simulink model "ROPOD_Control_WheelsRL_Code_GEN"  (R2020b)
settings: Solver=VariableStepAuto  StartTime=0.0  StopTime=10.0  RelTol=1e-3
values from neighbouring files (symbols this model uses):
  FFtheta_intia = 0    [init_model.m]
  FFxy_mass = 0*80    (= 0)    [init_model.m]
  I_fhz_ddelta_cntr = 0    [init_model.m]
  I_fhz_dtheta_cntr = 0.3    [init_model.m]
  I_fhz_dxdy_cntr = 0.25    [init_model.m]
  K_gain_ddelta_cntr = 0.2    [init_model.m]
  K_gain_dtheta_cntr = 150    [init_model.m]
  K_gain_dxdy_cntr = 200    [init_model.m]
  LL_wp_fhz_ddelta_cntr = 10    [init_model.m]
  LL_wp_fhz_dtheta_cntr = 20    [init_model.m]
  LL_wp_fhz_dxdy_cntr = 20    [init_model.m]
  LL_wz_fhz_ddelta_cntr = 2    [init_model.m]
  LL_wz_fhz_dtheta_cntr = 20    [init_model.m]
  LL_wz_fhz_dxdy_cntr = 20    [init_model.m]
  LPF_fhz_ddelta_cntr = 10    [init_model.m]
  LPF_fhz_ddelta_meas = 50    [init_model.m]
  LPF_fhz_dtheta_cntr = 100    [init_model.m]
  LPF_fhz_dvarphi_meas = 50    [init_model.m]
  LPF_fhz_dxdy_cntr = 100    [init_model.m]
  max_hw_tau = 7.0    (= 7)    [init_model.m]
  max_ropod_acc_theta = 1.6    [init_model.m]
  max_ropod_acc_xy = 2.0    (= 2)    [init_model.m]
  max_ropod_sw_force = 500    [init_model.m]
  max_ropod_sw_tau = 250    [init_model.m]
  max_ropod_vel_theta = 1.6    [init_model.m]
  max_ropod_vel_xy = 2.0    (= 2)    [init_model.m]
  max_sw_current = 10    [init_model.m]
  Nwheels = 4    [Jqwl_numeric_function.m]    (also in S_matrix.m; extract_kinmodel_parameters.m; init_model.m; tau_optimal_dist_vec_fun.m)
  pivot_offs_sws = [3.835 3.465 2.059 0.357]    [init_model.m]
  ropod_kinmodel_pv = struct2array(ropod_kinmodel_param)    [set_ropod_KinModparams.m]
  SW_COM1_ENABLE1 = hex2dec('0001')    [init_model.m]
  SW_COM1_ENABLE2 = hex2dec('0002')    [init_model.m]
  SW_COM1_MODE_TORQUE = bitshift(hex2dec('0000'),2)    [init_model.m]
  SW_COM1_MODE_VELOCITY = bitshift(hex2dec('0002'),2)    [init_model.m]
  SW_COM1_USE_TS = hex2dec('8000')    [init_model.m]
  Tinit = 0*Tslot    [init_model.m]
  Ts = 0.001    [init_model.m]
undefined symbols (not defined in the file or in its folder): AgentNumber, DiscIntNeverNeededParam, flock_FFtheta_friction, flock_FFxy_friction, I_fhz_dtheta_flock_cntr, I_fhz_dvarphi_cntr, I_fhz_dxdy_flock_cntr, K_gain_dtheta_flock_cntr, K_gain_dvarphi_cntr, K_gain_dxdy_flock_cntr, LL_wp_fhz_dtheta_flock_cntr, LL_wp_fhz_dvarphi_cntr, LL_wp_fhz_dxdy_flock_cntr, LL_wz_fhz_dtheta_flock_cntr, LL_wz_fhz_dvarphi_cntr, LL_wz_fhz_dxdy_flock_cntr, LPF_fhz_dtheta_flock_cntr, LPF_fhz_dvarphi_cntr, LPF_fhz_dxdy_flock_cntr, max_flock_acc_theta, max_flock_acc_xy, max_flock_vel_theta, max_flock_vel_xy, Nagents, ropod_position_inflock, sw_tau_2_current, Tsflck
libraries: simulink x62, pid_lib x60, cstblocks x54, dspsigops x24, SOEM_EtherCAT_Lib x5, dspnetwork x4
(part 10 of 11)

== system ROPOD_Control_WheelsRL_Code_GEN/RopodTorqueDistribution_/wheel vel cntr/Wheels Velocity controller/G_I_LL_LPF Controller7/Shapeit Integrator (Tustin) ==
  In : Inport
  I_fhz : Inport  Port=2
  reset : Inport  Port=3
  Constant : Constant  Value=0
  Constant4 : Constant
  Constant5 : Constant  Value=0
  Gain2 : Gain  Gain=2*pi
  PID Controller3 : pid_lib/PID Controller  Controller=PID  Form=Parallel  TimeDomain=Discrete-time  UseExternalTs=off  SampleTime=Ts  IntegratorMethod=Trapezoidal  FilterMethod=Trapezoidal  ControllerParametersSource=external  P=0.4  I=0.4*2*pi*3  D=0  UseFilter=on  N=100  TunerSelectOption=Transfer Function Based (PID Tuner App)  InitialConditionSource=internal  InitialConditionForIntegrator=0  InitialConditionForFilter=0  DifferentiatorICPrevScaledInput=0  ExternalReset=level  TrackingMode=off  Kt=1  LimitOutput=on  SatLimitsSource=internal  UpperSaturationLimit=max_hw_tau  LowerSaturationLimit=-max_hw_tau  LinearizeAsGain=on  AntiWindupMode=clamping  Kb=1  POutMin=[]  POutMax=[]  IOutMin=[]  IOutMax=[]  DOutMin=[]  DOutMax=[]  NOutMin=[]  NOutMax=[]  SumOutMin=[]  SumOutMax=[]  SaturationOutMin=[]  SaturationOutMax=[]  PParamMin=[]  PParamMax=[]  IParamMin=[]  IParamMax=[]  DParamMin=[]  DParamMax=[]  NParamMin=[]  NParamMax=[]  KbParamMin=[]  KbParamMax=[]  KtParamMin=[]  KtParamMax=[]  KbOutMin=[]  KbOutMax=[]  KtOutMin=[]  KtOutMax=[]  IntegratorOutMin=[]  IntegratorOutMax=[]  FilterOutMin=[]  FilterOutMax=[]  SumI1OutMin=[]  SumI1OutMax=[]  SumI2OutMin=[]  SumI2OutMax=[]  SumI3OutMin=[]  SumI3OutMax=[]  SumI4OutMin=[]  SumI4OutMax=[]  SumDOutMin=[]  SumDOutMax=[]  DifferentiatorOutMin=[]  DifferentiatorOutMax=[]  FilterDiffOutCoefMin=[]  FilterDiffOutCoefMax=[]  ReciprocalOutMin=[]  ReciprocalOutMax=[]  SumDenOutMin=[]  SumDenOutMax=[]  SumNumOutMin=[]  SumNumOutMax=[]  DivideOutMin=[]  DivideOutMax=[]  UdiffTsProdOutMin=[]  UdiffTsProdOutMax=[]  NTsProdOutMin=[]  NTsProdOutMax=[]  UintegralTsProdOutMin=[]  UintegralTsProdOutMax=[]  UngainTsProdOutMin=[]  UngainTsProdOutMax=[]  IntegratorContinuousStateAttributes=''  IntegratorStateMustResolveToSignalObject=off  IntegratorRTWStateStorageClass=Auto  FilterContinuousStateAttributes=''  FilterStateMustResolveToSignalObject=off  FilterRTWStateStorageClass=Auto  ParallelPVariant=ExternalParameters  IdealPVariant=Disabled  IVariant=ExternalParameters  DVariant=ExternalParameters  IntegratorVariant=Discrete  SatVariant=Enabled  AWVariant=DiscClampingParallel  PCopyVariant=Disabled  TRVariant=Disabled  FdbkBlocksVariant=Feedback  IdealPFdbkVariant=Passthrough  SatFdbkVariant=Passthrough  DerivativeFilterVariant=TrapezoidalFilter  NVariant=ExternalParameters  NCopyVariant=ExternalParameters  FilterICVariant=InternalICsFilter  IntegratorICVariant=InternalICs  ExternalResetVariant=ExternalReset  TRSumVariant=Passthrough  SumFdbkVariant=Enabled  SumVariant=Sum_PID  TsampFilterVariant=InternalTs  TsampNgainVariant=Passthrough  TsampIntegralVariant=Passthrough  ExternalSaturationOutDataTypeStr=Inherit: Same as second input
  Product4 : Product
  Out : Outport  VectorParamsAs1DForOutWhenUnconnected=off
  wires:
  Constant/1 -> PID Controller3/4
  Constant5/1 -> PID Controller3/5
  Constant4/1 -> PID Controller3/2, Product4/1
  In/1 -> PID Controller3/1
  PID Controller3/1 -> Out/1
  Gain2/1 -> PID Controller3/3
  reset/1 -> PID Controller3/6
  Product4/1 -> Gain2/1
  I_fhz/1 -> Product4/2

== system ROPOD_Control_WheelsRL_Code_GEN/RopodTorqueDistribution_/wheel vel cntr/Wheels Velocity controller/G_I_LL_LPF Controller7/Shapeit Lead-Lag (Tustin) ==
  In : Inport
  fz : Inport  Port=2
  fp : Inport  Port=3
  Add : Sum  Inputs=+-
  Constant1 : Constant
  Constant2 : Constant  Value=0
  Constant4 : Constant
  Divide : Product  Inputs=*/
  Divide1 : Product  Inputs=/*
  Gain1 : Gain  Gain=2*pi
  Gain2 : Gain  Gain=2*pi
  PID Controller3 : pid_lib/PID Controller  Controller=PID  Form=Parallel  TimeDomain=Discrete-time  UseExternalTs=off  SampleTime=Ts  IntegratorMethod=Trapezoidal  FilterMethod=Trapezoidal  ControllerParametersSource=external  P=0.4  I=0.4*2*pi*3  D=0  UseFilter=on  N=100  TunerSelectOption=Transfer Function Based (PID Tuner App)  InitialConditionSource=internal  InitialConditionForIntegrator=0  InitialConditionForFilter=0  DifferentiatorICPrevScaledInput=0  ExternalReset=none  TrackingMode=off  Kt=1  LimitOutput=off  SatLimitsSource=internal  UpperSaturationLimit=max_hw_tau  LowerSaturationLimit=-max_hw_tau  LinearizeAsGain=on  AntiWindupMode=clamping  Kb=1  POutMin=[]  POutMax=[]  IOutMin=[]  IOutMax=[]  DOutMin=[]  DOutMax=[]  NOutMin=[]  NOutMax=[]  SumOutMin=[]  SumOutMax=[]  SaturationOutMin=[]  SaturationOutMax=[]  PParamMin=[]  PParamMax=[]  IParamMin=[]  IParamMax=[]  DParamMin=[]  DParamMax=[]  NParamMin=[]  NParamMax=[]  KbParamMin=[]  KbParamMax=[]  KtParamMin=[]  KtParamMax=[]  KbOutMin=[]  KbOutMax=[]  KtOutMin=[]  KtOutMax=[]  IntegratorOutMin=[]  IntegratorOutMax=[]  FilterOutMin=[]  FilterOutMax=[]  SumI1OutMin=[]  SumI1OutMax=[]  SumI2OutMin=[]  SumI2OutMax=[]  SumI3OutMin=[]  SumI3OutMax=[]  SumI4OutMin=[]  SumI4OutMax=[]  SumDOutMin=[]  SumDOutMax=[]  DifferentiatorOutMin=[]  DifferentiatorOutMax=[]  FilterDiffOutCoefMin=[]  FilterDiffOutCoefMax=[]  ReciprocalOutMin=[]  ReciprocalOutMax=[]  SumDenOutMin=[]  SumDenOutMax=[]  SumNumOutMin=[]  SumNumOutMax=[]  DivideOutMin=[]  DivideOutMax=[]  UdiffTsProdOutMin=[]  UdiffTsProdOutMax=[]  NTsProdOutMin=[]  NTsProdOutMax=[]  UintegralTsProdOutMin=[]  UintegralTsProdOutMax=[]  UngainTsProdOutMin=[]  UngainTsProdOutMax=[]  IntegratorContinuousStateAttributes=''  IntegratorStateMustResolveToSignalObject=off  IntegratorRTWStateStorageClass=Auto  FilterContinuousStateAttributes=''  FilterStateMustResolveToSignalObject=off  FilterRTWStateStorageClass=Auto  ParallelPVariant=ExternalParameters  IdealPVariant=Disabled  IVariant=ExternalParameters  DVariant=ExternalParameters  IntegratorVariant=Discrete  SatVariant=Disabled  AWVariant=Passthrough  PCopyVariant=Disabled  TRVariant=Disabled  FdbkBlocksVariant=Forward  IdealPFdbkVariant=Disabled  SatFdbkVariant=Disabled  DerivativeFilterVariant=TrapezoidalFilter  NVariant=ExternalParameters  NCopyVariant=ExternalParameters  FilterICVariant=InternalICsFilter  IntegratorICVariant=InternalICs  ExternalResetVariant=Disabled  TRSumVariant=Passthrough  SumFdbkVariant=Disabled  SumVariant=Sum_PID  TsampFilterVariant=InternalTs  TsampNgainVariant=Passthrough  TsampIntegralVariant=Passthrough  ExternalSaturationOutDataTypeStr=Inherit: Same as second input
  Out : Outport  VectorParamsAs1DForOutWhenUnconnected=off
  wires:
  Divide1/1 -> PID Controller3/4
  Add/1 -> Divide1/2
  Constant1/1 -> Add/1
  Divide/1 -> Add/2
  Gain2/1 -> Divide/1, Divide1/1
  Constant2/1 -> PID Controller3/3
  Gain1/1 -> Divide/2, PID Controller3/5
  fp/1 -> Gain1/1
  fz/1 -> Gain2/1
  PID Controller3/1 -> Out/1
  In/1 -> PID Controller3/1
  Constant4/1 -> PID Controller3/2

== system ROPOD_Control_WheelsRL_Code_GEN/RopodTorqueDistribution_/wheel vel cntr/Wheels Velocity controller/G_I_LL_LPF Controller8/Shapeit Integrator (Tustin) ==
  In : Inport
  I_fhz : Inport  Port=2
  reset : Inport  Port=3
  Constant : Constant  Value=0
  Constant4 : Constant
  Constant5 : Constant  Value=0
  Gain2 : Gain  Gain=2*pi
  PID Controller3 : pid_lib/PID Controller  Controller=PID  Form=Parallel  TimeDomain=Discrete-time  UseExternalTs=off  SampleTime=Ts  IntegratorMethod=Trapezoidal  FilterMethod=Trapezoidal  ControllerParametersSource=external  P=0.4  I=0.4*2*pi*3  D=0  UseFilter=on  N=100  TunerSelectOption=Transfer Function Based (PID Tuner App)  InitialConditionSource=internal  InitialConditionForIntegrator=0  InitialConditionForFilter=0  DifferentiatorICPrevScaledInput=0  ExternalReset=level  TrackingMode=off  Kt=1  LimitOutput=on  SatLimitsSource=internal  UpperSaturationLimit=max_hw_tau  LowerSaturationLimit=-max_hw_tau  LinearizeAsGain=on  AntiWindupMode=clamping  Kb=1  POutMin=[]  POutMax=[]  IOutMin=[]  IOutMax=[]  DOutMin=[]  DOutMax=[]  NOutMin=[]  NOutMax=[]  SumOutMin=[]  SumOutMax=[]  SaturationOutMin=[]  SaturationOutMax=[]  PParamMin=[]  PParamMax=[]  IParamMin=[]  IParamMax=[]  DParamMin=[]  DParamMax=[]  NParamMin=[]  NParamMax=[]  KbParamMin=[]  KbParamMax=[]  KtParamMin=[]  KtParamMax=[]  KbOutMin=[]  KbOutMax=[]  KtOutMin=[]  KtOutMax=[]  IntegratorOutMin=[]  IntegratorOutMax=[]  FilterOutMin=[]  FilterOutMax=[]  SumI1OutMin=[]  SumI1OutMax=[]  SumI2OutMin=[]  SumI2OutMax=[]  SumI3OutMin=[]  SumI3OutMax=[]  SumI4OutMin=[]  SumI4OutMax=[]  SumDOutMin=[]  SumDOutMax=[]  DifferentiatorOutMin=[]  DifferentiatorOutMax=[]  FilterDiffOutCoefMin=[]  FilterDiffOutCoefMax=[]  ReciprocalOutMin=[]  ReciprocalOutMax=[]  SumDenOutMin=[]  SumDenOutMax=[]  SumNumOutMin=[]  SumNumOutMax=[]  DivideOutMin=[]  DivideOutMax=[]  UdiffTsProdOutMin=[]  UdiffTsProdOutMax=[]  NTsProdOutMin=[]  NTsProdOutMax=[]  UintegralTsProdOutMin=[]  UintegralTsProdOutMax=[]  UngainTsProdOutMin=[]  UngainTsProdOutMax=[]  IntegratorContinuousStateAttributes=''  IntegratorStateMustResolveToSignalObject=off  IntegratorRTWStateStorageClass=Auto  FilterContinuousStateAttributes=''  FilterStateMustResolveToSignalObject=off  FilterRTWStateStorageClass=Auto  ParallelPVariant=ExternalParameters  IdealPVariant=Disabled  IVariant=ExternalParameters  DVariant=ExternalParameters  IntegratorVariant=Discrete  SatVariant=Enabled  AWVariant=DiscClampingParallel  PCopyVariant=Disabled  TRVariant=Disabled  FdbkBlocksVariant=Feedback  IdealPFdbkVariant=Passthrough  SatFdbkVariant=Passthrough  DerivativeFilterVariant=TrapezoidalFilter  NVariant=ExternalParameters  NCopyVariant=ExternalParameters  FilterICVariant=InternalICsFilter  IntegratorICVariant=InternalICs  ExternalResetVariant=ExternalReset  TRSumVariant=Passthrough  SumFdbkVariant=Enabled  SumVariant=Sum_PID  TsampFilterVariant=InternalTs  TsampNgainVariant=Passthrough  TsampIntegralVariant=Passthrough  ExternalSaturationOutDataTypeStr=Inherit: Same as second input
  Product4 : Product
  Out : Outport  VectorParamsAs1DForOutWhenUnconnected=off
  wires:
  I_fhz/1 -> Product4/2
  Product4/1 -> Gain2/1
  reset/1 -> PID Controller3/6
  Gain2/1 -> PID Controller3/3
  PID Controller3/1 -> Out/1
  In/1 -> PID Controller3/1
  Constant4/1 -> Product4/1, PID Controller3/2
  Constant5/1 -> PID Controller3/5
  Constant/1 -> PID Controller3/4

== system ROPOD_Control_WheelsRL_Code_GEN/RopodTorqueDistribution_/wheel vel cntr/Wheels Velocity controller/G_I_LL_LPF Controller8/Shapeit Lead-Lag (Tustin) ==
  In : Inport
  fz : Inport  Port=2
  fp : Inport  Port=3
  Add : Sum  Inputs=+-
  Constant1 : Constant
  Constant2 : Constant  Value=0
  Constant4 : Constant
  Divide : Product  Inputs=*/
  Divide1 : Product  Inputs=/*
  Gain1 : Gain  Gain=2*pi
  Gain2 : Gain  Gain=2*pi
  PID Controller3 : pid_lib/PID Controller  Controller=PID  Form=Parallel  TimeDomain=Discrete-time  UseExternalTs=off  SampleTime=Ts  IntegratorMethod=Trapezoidal  FilterMethod=Trapezoidal  ControllerParametersSource=external  P=0.4  I=0.4*2*pi*3  D=0  UseFilter=on  N=100  TunerSelectOption=Transfer Function Based (PID Tuner App)  InitialConditionSource=internal  InitialConditionForIntegrator=0  InitialConditionForFilter=0  DifferentiatorICPrevScaledInput=0  ExternalReset=none  TrackingMode=off  Kt=1  LimitOutput=off  SatLimitsSource=internal  UpperSaturationLimit=max_hw_tau  LowerSaturationLimit=-max_hw_tau  LinearizeAsGain=on  AntiWindupMode=clamping  Kb=1  POutMin=[]  POutMax=[]  IOutMin=[]  IOutMax=[]  DOutMin=[]  DOutMax=[]  NOutMin=[]  NOutMax=[]  SumOutMin=[]  SumOutMax=[]  SaturationOutMin=[]  SaturationOutMax=[]  PParamMin=[]  PParamMax=[]  IParamMin=[]  IParamMax=[]  DParamMin=[]  DParamMax=[]  NParamMin=[]  NParamMax=[]  KbParamMin=[]  KbParamMax=[]  KtParamMin=[]  KtParamMax=[]  KbOutMin=[]  KbOutMax=[]  KtOutMin=[]  KtOutMax=[]  IntegratorOutMin=[]  IntegratorOutMax=[]  FilterOutMin=[]  FilterOutMax=[]  SumI1OutMin=[]  SumI1OutMax=[]  SumI2OutMin=[]  SumI2OutMax=[]  SumI3OutMin=[]  SumI3OutMax=[]  SumI4OutMin=[]  SumI4OutMax=[]  SumDOutMin=[]  SumDOutMax=[]  DifferentiatorOutMin=[]  DifferentiatorOutMax=[]  FilterDiffOutCoefMin=[]  FilterDiffOutCoefMax=[]  ReciprocalOutMin=[]  ReciprocalOutMax=[]  SumDenOutMin=[]  SumDenOutMax=[]  SumNumOutMin=[]  SumNumOutMax=[]  DivideOutMin=[]  DivideOutMax=[]  UdiffTsProdOutMin=[]  UdiffTsProdOutMax=[]  NTsProdOutMin=[]  NTsProdOutMax=[]  UintegralTsProdOutMin=[]  UintegralTsProdOutMax=[]  UngainTsProdOutMin=[]  UngainTsProdOutMax=[]  IntegratorContinuousStateAttributes=''  IntegratorStateMustResolveToSignalObject=off  IntegratorRTWStateStorageClass=Auto  FilterContinuousStateAttributes=''  FilterStateMustResolveToSignalObject=off  FilterRTWStateStorageClass=Auto  ParallelPVariant=ExternalParameters  IdealPVariant=Disabled  IVariant=ExternalParameters  DVariant=ExternalParameters  IntegratorVariant=Discrete  SatVariant=Disabled  AWVariant=Passthrough  PCopyVariant=Disabled  TRVariant=Disabled  FdbkBlocksVariant=Forward  IdealPFdbkVariant=Disabled  SatFdbkVariant=Disabled  DerivativeFilterVariant=TrapezoidalFilter  NVariant=ExternalParameters  NCopyVariant=ExternalParameters  FilterICVariant=InternalICsFilter  IntegratorICVariant=InternalICs  ExternalResetVariant=Disabled  TRSumVariant=Passthrough  SumFdbkVariant=Disabled  SumVariant=Sum_PID  TsampFilterVariant=InternalTs  TsampNgainVariant=Passthrough  TsampIntegralVariant=Passthrough  ExternalSaturationOutDataTypeStr=Inherit: Same as second input
  Out : Outport  VectorParamsAs1DForOutWhenUnconnected=off
  wires:
  Constant4/1 -> PID Controller3/2
  In/1 -> PID Controller3/1
  PID Controller3/1 -> Out/1
  fz/1 -> Gain2/1
  fp/1 -> Gain1/1
  Gain1/1 -> PID Controller3/5, Divide/2
  Constant2/1 -> PID Controller3/3
  Gain2/1 -> Divide1/1, Divide/1
  Divide/1 -> Add/2
  Constant1/1 -> Add/1
  Add/1 -> Divide1/2
  Divide1/1 -> PID Controller3/4

== matlab function ROPOD_Control_WheelsRL_Code_GEN/RopodTorqueDistribution/ROPOD 4SW/ROPOD_4Wheel_sens_own_vel_filter/Glitch removal + LP filter4/Remove_glitches1 ==
  data: vel input; Ts input; encoder input; encoder_out output
function encoder_out  = remove_glitches(vel, Ts, encoder)

persistent last_valid_encoder;
persistent invalid_cnt;

if(isempty(last_valid_encoder))
    last_valid_encoder = encoder;
    invalid_cnt = 0;
end

if abs( (last_valid_encoder-encoder)/Ts ) > 50 % maximum expected velocity rad/sec (2.5 m/s)
    encoder_out = last_valid_encoder + vel*Ts;    
    invalid_cnt = invalid_cnt +1;
else
    encoder_out = encoder;
end

if invalid_cnt>1 
    invalid_cnt = 0;
    encoder_out = encoder;
end

last_valid_encoder = encoder_out;

== matlab function ROPOD_Control_WheelsRL_Code_GEN/RopodTorqueDistribution/ROPOD 4SW/ROPOD_4Wheel_sens_own_vel_filter/Glitch removal + LP filter5/Remove_glitches1 ==
  data: vel input; Ts input; encoder input; encoder_out output
function encoder_out  = remove_glitches(vel, Ts, encoder)

persistent last_valid_encoder;
persistent invalid_cnt;

if(isempty(last_valid_encoder))
    last_valid_encoder = encoder;
    invalid_cnt = 0;
end

if abs( (last_valid_encoder-encoder)/Ts ) > 50 % maximum expected velocity rad/sec (2.5 m/s)
    encoder_out = last_valid_encoder + vel*Ts;    
    invalid_cnt = invalid_cnt +1;
else
    encoder_out = encoder;
end

if invalid_cnt>1 
    invalid_cnt = 0;
    encoder_out = encoder;
end

last_valid_encoder = encoder_out;

== matlab function ROPOD_Control_WheelsRL_Code_GEN/From ROS (Parameters and topics)/rot_matrix2 ==
  data: dqr_glb input; theta input; dqr_loc output
function dqr_loc   = zrot(dqr_glb, theta)
%ROPOD_JACOBIAN Summary of this function goes here
%   Detailed explanation goes here


dqr_loc = [  cos(-theta) -sin(-theta) 0; 
            sin(-theta)  cos(-theta) 0;
                    0             0  1]*dqr_glb;
end

== matlab function ROPOD_Control_WheelsRL_Code_GEN/RopodTorqueDistribution/ROPOD 4SW/ROPOD_4Wheel_sens_own_vel_filter/Glitch removal + LP filter6/Remove_glitches1 ==
  data: vel input; Ts input; encoder input; encoder_out output
function encoder_out  = remove_glitches(vel, Ts, encoder)

persistent last_valid_encoder;
persistent invalid_cnt;

if(isempty(last_valid_encoder))
    last_valid_encoder = encoder;
    invalid_cnt = 0;
end

if abs( (last_valid_encoder-encoder)/Ts ) > 50 % maximum expected velocity rad/sec (2.5 m/s)
    encoder_out = last_valid_encoder + vel*Ts;    
    invalid_cnt = invalid_cnt +1;
else
    encoder_out = encoder;
end

if invalid_cnt>1 
    invalid_cnt = 0;
    encoder_out = encoder;
end

last_valid_encoder = encoder_out;

== matlab function ROPOD_Control_WheelsRL_Code_GEN/RopodTorqueDistribution/ROPOD 4SW/ROPOD_4Wheel_sens_own_vel_filter/Glitch removal + LP filter7/Remove_glitches1 ==
  data: vel input; Ts input; encoder input; encoder_out output
function encoder_out  = remove_glitches(vel, Ts, encoder)

persistent last_valid_encoder;
persistent invalid_cnt;

if(isempty(last_valid_encoder))
    last_valid_encoder = encoder;
    invalid_cnt = 0;
end

if abs( (last_valid_encoder-encoder)/Ts ) > 50 % maximum expected velocity rad/sec (2.5 m/s)
    encoder_out = last_valid_encoder + vel*Ts;    
    invalid_cnt = invalid_cnt +1;
else
    encoder_out = encoder;
end

if invalid_cnt>1 
    invalid_cnt = 0;
    encoder_out = encoder;
end

last_valid_encoder = encoder_out;

== matlab function ROPOD_Control_WheelsRL_Code_GEN/RopodTorqueDistribution/ROPOD 4SW/ROPOD_4Wheel_sens_own_vel_filter/Glitch removal + LP filter8/Remove_glitches1 ==
  data: vel input; Ts input; encoder input; encoder_out output
function encoder_out  = remove_glitches(vel, Ts, encoder)

persistent last_valid_encoder;
persistent invalid_cnt;

if(isempty(last_valid_encoder))
    last_valid_encoder = encoder;
    invalid_cnt = 0;
end

if abs( (last_valid_encoder-encoder)/Ts ) > 50 % maximum expected velocity rad/sec (2.5 m/s)
    encoder_out = last_valid_encoder + vel*Ts;    
    invalid_cnt = invalid_cnt +1;
else
    encoder_out = encoder;
end

if invalid_cnt>1 
    invalid_cnt = 0;
    encoder_out = encoder;
end

last_valid_encoder = encoder_out;

== matlab function ROPOD_Control_WheelsRL_Code_GEN/RopodTorqueDistribution/ROPOD 4SW/ROPOD_4Wheel_sens_own_vel_filter/Glitch removal + LP filter10/Remove_glitches1 ==
  data: vel input; Ts input; encoder input; encoder_out output
function encoder_out  = remove_glitches(vel, Ts, encoder)

persistent last_valid_encoder;
persistent invalid_cnt;

if(isempty(last_valid_encoder))
    last_valid_encoder = encoder;
    invalid_cnt = 0;
end

if abs( (last_valid_encoder-encoder)/Ts ) > 50 % maximum expected velocity rad/sec (2.5 m/s)
    encoder_out = last_valid_encoder + vel*Ts;    
    invalid_cnt = invalid_cnt +1;
else
    encoder_out = encoder;
end

if invalid_cnt>1 
    invalid_cnt = 0;
    encoder_out = encoder;
end

last_valid_encoder = encoder_out;

== matlab function ROPOD_Control_WheelsRL_Code_GEN/RopodTorqueDistribution/ROPOD 4SW/ROPOD_4Wheel_sens_own_vel_filter/Glitch removal + LP filter11/Remove_glitches1 ==
  data: vel input; Ts input; encoder input; encoder_out output
function encoder_out  = remove_glitches(vel, Ts, encoder)

persistent last_valid_encoder;
persistent invalid_cnt;

if(isempty(last_valid_encoder))
    last_valid_encoder = encoder;
    invalid_cnt = 0;
end

if abs( (last_valid_encoder-encoder)/Ts ) > 50 % maximum expected velocity rad/sec (2.5 m/s)
    encoder_out = last_valid_encoder + vel*Ts;    
    invalid_cnt = invalid_cnt +1;
else
    encoder_out = encoder;
end

if invalid_cnt>1 
    invalid_cnt = 0;
    encoder_out = encoder;
end

last_valid_encoder = encoder_out;

== matlab function ROPOD_Control_WheelsRL_Code_GEN/RopodTorqueDistribution/ROPOD 4SW/ROPOD_4Wheel_sens_own_vel_filter/Glitch removal + LP filter9/Remove_glitches1 ==
  data: vel input; Ts input; encoder input; encoder_out output
function encoder_out  = remove_glitches(vel, Ts, encoder)

persistent last_valid_encoder;
persistent invalid_cnt;

if(isempty(last_valid_encoder))
    last_valid_encoder = encoder;
    invalid_cnt = 0;
end

if abs( (last_valid_encoder-encoder)/Ts ) > 50 % maximum expected velocity rad/sec (2.5 m/s)
    encoder_out = last_valid_encoder + vel*Ts;    
    invalid_cnt = invalid_cnt +1;
else
    encoder_out = encoder;
end

if invalid_cnt>1 
    invalid_cnt = 0;
    encoder_out = encoder;
end

last_valid_encoder = encoder_out;

== matlab function ROPOD_Control_WheelsRL_Code_GEN/FlockController/InverseKinematicsFlock ==
  data: enable input; invMG output; G output; enable_agents input; position_agents input
function [invMG , G]  = inverseKinematicsFlock(enable, enable_agents, position_agents)


Nagents = length(enable_agents);

%% First compute the matrix from v to W_wh

% Gi = zeros([2 3]);
G = zeros(3*Nagents,3);
M = zeros(3*Nagents,3*Nagents);
invMG = zeros(3,3*Nagents);
if (enable)
    for i=1:Nagents
        % To obtain ropod velocities in Flock coordinates, add vectors of
        % translations and movement due to flock angular velocity.
        Gi = [1  0 -position_agents(2,i);
            0  1  position_agents(1,i)
            0  0  1];
        
        % Rotation to obtain pivot Wi velocity vector in wheel coordinates
        Gi(1:2,1:3) = [   cos(-position_agents(3,i))     -sin(-position_agents(3,i)); ...
            sin(-position_agents(3,i))     cos(-position_agents(3,i))]*Gi(1:2,1:3);
        
        G(3*(i-1)+1:3*i,:) = Gi;
        M(3*(i-1)+1:3*i,3*(i-1)+1:3*i)=diag([enable_agents(i) enable_agents(i) enable_agents(i)]);
    end
    
    MG = (M*G);
    invMG = pinv(MG);
end
end

== matlab function ROPOD_Control_WheelsRL_Code_GEN/FlockController/Deserialization ==
  data: ext_agents_configuration input; enable_ext_agents output; position_ext_agents output; local_velocity_ext_agents output; constraints_ext_agents output
function [enable_ext_agents, position_ext_agents, local_velocity_ext_agents, constraints_ext_agents ] = deserializeFlockData(ext_agents_configuration)

size_pa = 1+3+3+8;
Nagents = (length(ext_agents_configuration)/size_pa) + 1; %

enable_ext_agents = zeros(1,Nagents-1);
position_ext_agents = zeros(3,Nagents-1);
local_velocity_ext_agents = zeros(3,Nagents-1);
constraints_ext_agents = zeros(4*2,Nagents-1);

for i_cnt = 1:(Nagents-1)
    enable_ext_agents(i_cnt) = ext_agents_configuration((Nagents-1)*(i_cnt-1)+1);
    position_ext_agents(:,i_cnt) = ext_agents_configuration((Nagents-1)*(i_cnt-1)+(2:4));
    local_velocity_ext_agents(:,i_cnt) = ext_agents_configuration((Nagents-1)*(i_cnt-1)+(5:7));
    constraints_ext_agents(:,i_cnt) = ext_agents_configuration((Nagents-1)*(i_cnt-1)+(8:size_pa));
end

== matlab function ROPOD_Control_WheelsRL_Code_GEN/FlockController/Optimization Matrices Calculation ==
  data: enable_agents input; A_agents output; AR_agents output; bR_agents output; position_agents input; constraints_agents input
function [A_agents, AR_agents, bR_agents] = computeOptMatrices(enable_agents, position_agents, constraints_agents )

Nagents = length(enable_agents); %

A_agents = zeros(3,3,Nagents);
AR_agents = zeros(6,3,Nagents); % TODO: 4 lines +2 of ropods
bR_agents = zeros(6,1,Nagents);

for i_agnt = 1:Nagents
    x_agnt = position_agents(1,i_agnt);
    x_agnt_torque = x_agnt;
    y_agnt = position_agents(2,i_agnt);
    y_agnt_torque = y_agnt;
    th_agnt = position_agents(3,i_agnt);
    
    % For now no torque is assigned to ropods.
    % On one hand it is not desired, on the other,
    % when arm aproaches 0, more torque is assigned and
    % there is a singularity
    tau_max_ropod = 0;
    if (x_agnt_torque==0)
        x_agnt_torque = 0.1;
    elseif(abs(x_agnt_torque) < 0.1)
        x_agnt_torque = 0.1*sign(x_agnt_torque);
    end
    
    if (y_agnt_torque==0)
        y_agnt_torque = 0.1;
    elseif(abs(y_agnt_torque) < 0.1)
        y_agnt_torque = 0.1*sign(y_agnt_torque);
    end    
    
    A_agents(:,:,i_agnt) = ...
        [
                                          cos(th_agnt)                                    sin(th_agnt)    1/y_agnt_torque;
                                          sin(th_agnt)                                    cos(th_agnt)   -1/x_agnt_torque;
        -( y_agnt*cos(th_agnt) + x_agnt*sin(th_agnt) )   ( x_agnt*cos(th_agnt) - y_agnt*sin(th_agnt) )           1;
        ];
    
    
   
    AgntConst = zeros(4,2);
    for i_agcnst = 1:4 % constraints of a single agent
        AgntConst(i_agcnst,:) = constraints_agents(2*(i_agcnst-1)+1 : 2*(i_agcnst-1)+2 ,i_agnt);      
    end

    AR_agents(:,:,i_agnt) = ...
        [
        [AgntConst(1,2)-AgntConst(2,2) AgntConst(2,1)-AgntConst(1,1) 0];
        [AgntConst(2,2)-AgntConst(3,2) AgntConst(3,1)-AgntConst(2,1) 0];
        [AgntConst(3,2)-AgntConst(4,2) AgntConst(4,1)-AgntConst(3,1) 0];
        [AgntConst(4,2)-AgntConst(1,2) AgntConst(1,1)-AgntConst(4,1) 0];
        [0 0 1];
        [0 0 -1];
        ];
    % prevent trivial problem leading to incorrect solution
    if(AR_agents(1:4,:,i_agnt) ==  zeros(4,3))
        small_number = 0.1;
        AR_agents(1:4,:,i_agnt) =   [   -small_number -small_number 0;
                                         small_number -small_number 0;
                                         small_number  small_number 0;
                                        -small_number  small_number 0;
                                    ];                 
    end
    
    bR_agents(:,:,i_agnt) = ...
        [
        -(AgntConst(1,1)*AgntConst(2,2)-AgntConst(2,1)*AgntConst(1,2));
        -(AgntConst(2,1)*AgntConst(3,2)-AgntConst(3,1)*AgntConst(2,2));
        -(AgntConst(3,1)*AgntConst(4,2)-AgntConst(4,1)*AgntConst(3,2));
        -(AgntConst(4,1)*AgntConst(1,2)-AgntConst(1,1)*AgntConst(4,2));
        -tau_max_ropod;
        -tau_max_ropod; 
        ];
end

== matlab function ROPOD_Control_WheelsRL_Code_GEN/RopodTorqueDistribution/Torque distribution using pseudoinverse/Gl_matrices ==
  data: ropod_kinmodel_param_vec input; Gl output; delta input; Gtl output; GtSl output
function [Gl, Gtl, GtSl]   = G_matrices( ropod_kinmodel_param_vec, delta)
%ROPOD_JACOBIAN Summary of this function goes here
%   Detailed explanation goes here


Gl    = Gl_matrix_wrapper(ropod_kinmodel_param_vec, delta);
Gtl   = Gl.';
GtSl  = Gtl*S_matrix();
end

== matlab function ROPOD_Control_WheelsRL_Code_GEN/MATLAB Function ==
  data: ext_agents_configuration_ini input; out_ext_agents_configuration output; message_in input; length_in input
function out_ext_agents_configuration = concatenate_agents_conf(ext_agents_configuration_ini, message_in, length_in)
size_ag_conf = 1+3+3+8;
Nagents = length(ext_agents_configuration_ini)/size_ag_conf +1;
% ext_agents_configuration_ini(1) - enabled
% ext_agents_configuration_ini(2:4) - relative position to bed's center
% ext_agents_configuration_ini(5:7) - local velocity
% ext_agents_configuration_ini(8:15) - 4 constraints points

% message_in(1) - agentNumber. By definition is from 2 to Nagents. 1 is reserved for coordinator
% message_in(2:end) - agent configuration

persistent ext_agents_configuration
if isempty(ext_agents_configuration)
    ext_agents_configuration = ext_agents_configuration_ini;
end

agentNumber = message_in(1);
if(length_in==(size_ag_conf+1) && agentNumber>=2 && agentNumber<=Nagents)
    i_agnt = agentNumber-1;
    ext_agents_configuration( (i_agnt-1)*size_ag_conf+1 : i_agnt*size_ag_conf) = message_in(2:end);
end


out_ext_agents_configuration = ext_agents_configuration;




end

== matlab function ROPOD_Control_WheelsRL_Code_GEN/RopodTorqueDistribution/wheel flip compensation/MATLAB Function1 ==
  data: tl input; tl_out output; tr input; ropod_kinmodel_param_vec input size=18; tr_out output; kmax input; sc output; Fthr input; tau_max input
function [tl_out,tr_out, sc] = fcn(tl, tr, ropod_kinmodel_param_vec, kmax, Fthr, tau_max)

[  rW1_1,rW1_2,rW1_3,rW1_4,rW2_1,rW2_2,rW2_3,rW2_4,...
    s_w,...
    d_w, ...
    CW1_1,CW1_2,CW1_3,CW1_4,CW2_1,CW2_2,CW2_3,CW2_4 ...
    ]= extract_kinmodel_parameters(ropod_kinmodel_param_vec);

Fxi = (tl/rW1_1+tr/rW1_2);
Fyi = (tr/rW1_2-tl/rW1_1)*(d_w/(2*s_w));
theta = atan2(Fyi,Fxi);

Fsize = abs(Fyi);
if Fsize> Fthr
   sc = (1+(kmax-1)*abs( sin(theta)) );
else
    sc = 1;
end

avg_t = (tr+tl)/2;
diff_t = (tr-tl)/2;
tl_out = avg_t-sc*diff_t;
tr_out = avg_t+sc*diff_t;

if(abs(tl_out)>tau_max && abs(tl_out)>abs(tr_out))
    sc = tau_max/abs(tl_out);
    tl_out = sc*tl_out;
    tr_out = sc*tr_out;
end

if(abs(tr_out)>tau_max && abs(tr_out)>abs(tl_out))
    sc = tau_max/abs(tr_out);
    tl_out = sc*tl_out;
    tr_out = sc*tr_out;
end

== matlab function ROPOD_Control_WheelsRL_Code_GEN/MATLAB Function1 ==
  data: AgentNumber input; WrenchAgent output; message_in input; length_msg input; dqAgent output
function [WrenchAgent, dqAgent] = concatenate_agents_conf(AgentNumber, message_in, length_msg)
Nagents = length(message_in)/3+1;

persistent WrenchAgent_
persistent dqAgent_

if isempty(WrenchAgent_)
    WrenchAgent_ = [0 0 0]';
    dqAgent_ = [0 0 0]';
end

if ( length_msg == 3*(Nagents-1)  && AgentNumber>=2 && AgentNumber<=Nagents)
    WrenchAgent_(1:3) = message_in(((AgentNumber-1)-1)*3+1:(AgentNumber-1)*3);
    dqAgent_(1:3) = message_in( ((AgentNumber-1)-1)*3+1+3*Nagents:(AgentNumber-1)*3 + 3*Nagents);
end

WrenchAgent = WrenchAgent_;
dqAgent = dqAgent_;



end

== matlab function ROPOD_Control_WheelsRL_Code_GEN/FlockController/Wrench Distributor ==
  data: wact input; is_coordinator input; Arow input; AR input; bR input; wR1 output; w_agents output; alpha output
function [wR1, w_agents, alpha] = DistributeWrenchOptimally(wact, is_coordinator, Arow, AR, bR)
%#codegen

Nagents = size(AR,3);
    if is_coordinator == 1  
        %% Function initalization
        % x = [wR1; ...; wRi; alpha]
        % wact = [Fx; Fy; \tau_z]
       
    %     useAlpha = 1;
    %     if useAlpha == 1
        %% Equalities
        Aeq = [zeros(3,3*Nagents) wact];
        beq = wact;
        % Aeq and beq might  be extended to include alpha ? (For which there no
        % equalities)

        %% Inequalities  
        A = zeros(2*(3*Nagents+1), Nagents*3+1);
        b = zeros(2*(3*Nagents+1), 1);

        % Put inequalities of each ropod into the master optimizer
        for iagent = 1:Nagents
            Aeq(:, 3*(iagent-1)+1:3*(iagent-1)+3) = Arow(:,:,iagent);
            A(6*(iagent-1)+1:6*(iagent-1)+6  ,  3*(iagent-1)+1:3*(iagent-1)+3) = AR(:,:,iagent);
            b(6*(iagent-1)+1:6*(iagent-1)+6) = bR(:,:,iagent);
        end
        
%         A(1:6, 1:3) = AR1;
%         b(1:6) = bR1;
%         
%         if Nagents == 2
%             A(7:12, 4:6) = AR2; % For 2 ropods
%             b(7:12) = bR2;
%         end

        % Inequalities for alpha
        A((Nagents*6)+1:(Nagents*6)+2, 3*Nagents+1) = [1; -1];
        b((Nagents*6)+1:(Nagents*6)+2) = [0; -1];

        H = eye(3*Nagents+1);
        H(3*Nagents+1, 3*Nagents+1) = 1;
        % Find the lower-triangular Cholesky decomposition of H.

        % We assume diagonal and square H;
        Linv = zeros(3*Nagents+1); 
        for icnt = 1:(3*Nagents+1)
            Linv(icnt,icnt) = 1/H(icnt,icnt); % equivalent to H = P^2H
        end        
        
    %     Linv = eye(3*Nagents+1);
        f = zeros(3*Nagents+1, 1);
        Fxmax = 425;
        Fymax = 1700;
        f(3*Nagents+1) = 0.5*(Fxmax^2+Fymax^2);
        x = zeros(3*Nagents+1,1);
        status = 0;
%         [x, status] = mpcqpsolver(Linv, f, A, b, Aeq, beq, false(Nagents*6+2, 1), mpcqpsolverOptions());
        [x, status] = mpcqpsolver(Linv, f, A, b, Aeq, beq, false(2*(3*Nagents+1), 1), mpcqpsolverOptions());
        if status <= 0
%             disp('Problem is not feasible!');
              wR1 = zeros(3,1);
              w_agents = zeros(3*(Nagents-1), 1);
              alpha = 1;
        else
            wR1 = x(1:3);
            if Nagents == 1
                w_agents = zeros(3, 1);
            else
                w_agents = x(4:Nagents*3);
            end
            alpha = x(Nagents*3 + 1);            
        end

    else
        wR1 = wact;
        w_agents = zeros(3*(Nagents-1), 1);
        alpha = 0;
    end
end

== matlab function ROPOD_Control_WheelsRL_Code_GEN/RopodTorqueDistribution/Torque distribution/Gl_matrices ==
  data: ropod_kinmodel_param_vec input; Gl output; delta input; Gtl output; GtSl output
function [Gl, Gtl, GtSl]   = G_matrices( ropod_kinmodel_param_vec, delta)
%ROPOD_JACOBIAN Summary of this function goes here
%   Detailed explanation goes here


Gl    = Gl_matrix_wrapper(ropod_kinmodel_param_vec, delta);
Gtl   = Gl.';
GtSl  = Gtl*S_matrix();
end

== matlab function ROPOD_Control_WheelsRL_Code_GEN/RopodTorqueDistribution/Torque distribution/platform_forces_2_tau_dist_optimal ==
  data: GtSl input; taubody input; ena_w input; Ttaud output; tau_max input; taubody_sc output
function [Ttaud, taubody_sc]   = Ttaud_optimal_vec( GtSl, taubody, ena_w , tau_max)
%#codegen

[Ttaud, taubody_sc]   = tau_optimal_dist_vec_fun( GtSl, taubody, ena_w, tau_max);

end

== matlab function ROPOD_Control_WheelsRL_Code_GEN/RopodTorqueDistribution/wheel flip compensation/MATLAB Function2 ==
  data: tl input; tl_out output; tr input; ropod_kinmodel_param_vec input size=18; tr_out output; kmax input; sc output; Fthr input; tau_max input
function [tl_out,tr_out, sc] = fcn(tl, tr, ropod_kinmodel_param_vec, kmax, Fthr, tau_max)

[  rW1_1,rW1_2,rW1_3,rW1_4,rW2_1,rW2_2,rW2_3,rW2_4,...
    s_w,...
    d_w, ...
    CW1_1,CW1_2,CW1_3,CW1_4,CW2_1,CW2_2,CW2_3,CW2_4 ...
    ]= extract_kinmodel_parameters(ropod_kinmodel_param_vec);

Fxi = (tl/rW1_1+tr/rW1_2);
Fyi = (tr/rW1_2-tl/rW1_1)*(d_w/(2*s_w));
theta = atan2(Fyi,Fxi);

Fsize = abs(Fyi);
if Fsize> Fthr
   sc = (1+(kmax-1)*abs( sin(theta)) );
else
    sc = 1;
end

avg_t = (tr+tl)/2;
diff_t = (tr-tl)/2;
tl_out = avg_t-sc*diff_t;
tr_out = avg_t+sc*diff_t;

if(abs(tl_out)>tau_max && abs(tl_out)>abs(tr_out))
    sc = tau_max/abs(tl_out);
    tl_out = sc*tl_out;
    tr_out = sc*tr_out;
end

if(abs(tr_out)>tau_max && abs(tr_out)>abs(tl_out))
    sc = tau_max/abs(tr_out);
    tl_out = sc*tl_out;
    tr_out = sc*tr_out;
end

== matlab function ROPOD_Control_WheelsRL_Code_GEN/RopodTorqueDistribution/wheel flip compensation/MATLAB Function3 ==
  data: tl input; tl_out output; tr input; ropod_kinmodel_param_vec input size=18; tr_out output; kmax input; sc output; Fthr input; tau_max input
function [tl_out,tr_out, sc] = fcn(tl, tr, ropod_kinmodel_param_vec, kmax, Fthr, tau_max)

[  rW1_1,rW1_2,rW1_3,rW1_4,rW2_1,rW2_2,rW2_3,rW2_4,...
    s_w,...
    d_w, ...
    CW1_1,CW1_2,CW1_3,CW1_4,CW2_1,CW2_2,CW2_3,CW2_4 ...
    ]= extract_kinmodel_parameters(ropod_kinmodel_param_vec);

Fxi = (tl/rW1_1+tr/rW1_2);
Fyi = (tr/rW1_2-tl/rW1_1)*(d_w/(2*s_w));
theta = atan2(Fyi,Fxi);

Fsize = abs(Fyi);
if Fsize> Fthr
   sc = (1+(kmax-1)*abs( sin(theta)) );
else
    sc = 1;
end

avg_t = (tr+tl)/2;
diff_t = (tr-tl)/2;
tl_out = avg_t-sc*diff_t;
tr_out = avg_t+sc*diff_t;

if(abs(tl_out)>tau_max && abs(tl_out)>abs(tr_out))
    sc = tau_max/abs(tl_out);
    tl_out = sc*tl_out;
    tr_out = sc*tr_out;
end

if(abs(tr_out)>tau_max && abs(tr_out)>abs(tl_out))
    sc = tau_max/abs(tr_out);
    tl_out = sc*tl_out;
    tr_out = sc*tr_out;
end

== matlab function ROPOD_Control_WheelsRL_Code_GEN/RopodTorqueDistribution/Torque distribution using pseudoinverse/platform_forces_2_tau_dist_optimal_pseudo_inverse ==
  data: GtSl input; taubody input; ena_w input; varphi_tau output; tau_max input; taubody_sc output
function [varphi_tau, taubody_sc]   = Ttaud_optimal_vec( GtSl, taubody, ena_w , tau_max)
%#codegen

Nwheels = 4;

% Optimization
M = eye(2*Nwheels);
for idx = 1:Nwheels
    M(2*(idx-1)+1,2*(idx-1)+1) = ena_w(idx);
    M(2*(idx-1)+2,2*(idx-1)+2) = ena_w(idx);
end
GM = GtSl*M;

varphi_tau_int = pinv(GM)*taubody;
varphi_tau_int_max = max(abs(varphi_tau_int));
 

if(varphi_tau_int_max > tau_max)
    taubody_sc = tau_max/varphi_tau_int_max;
else
    taubody_sc = 1.0;
end

varphi_tau = taubody_sc*varphi_tau_int;

end

== matlab function ROPOD_Control_WheelsRL_Code_GEN/RopodTorqueDistribution/Inverse Kinematics 4SW/Gl_matrix ==
  data: ropod_kinmodel_param_vec input; Gl output; delta input
function Gl = Gl_matrix_wrapper(ropod_kinmodel_param_vec, delta)

Gl = Gl_matrix_wrapper(ropod_kinmodel_param_vec, delta);

end

== matlab function ROPOD_Control_WheelsRL_Code_GEN/RopodTorqueDistribution_/Inverse Kinematics 4SW/Gl_matrix ==
  data: ropod_kinmodel_param_vec input; Gl output; delta input
function Gl = Gl_matrix_wrapper(ropod_kinmodel_param_vec, delta)

Gl = Gl_matrix_wrapper(ropod_kinmodel_param_vec, delta);

end

== matlab function ROPOD_Control_WheelsRL_Code_GEN/RopodTorqueDistribution/wheel flip compensation/MATLAB Function4 ==
  data: tl input; tl_out output; tr input; ropod_kinmodel_param_vec input size=18; tr_out output; kmax input; sc output; Fthr input; tau_max input
function [tl_out,tr_out, sc] = fcn(tl, tr, ropod_kinmodel_param_vec, kmax, Fthr, tau_max)

[  rW1_1,rW1_2,rW1_3,rW1_4,rW2_1,rW2_2,rW2_3,rW2_4,...
    s_w,...
    d_w, ...
    CW1_1,CW1_2,CW1_3,CW1_4,CW2_1,CW2_2,CW2_3,CW2_4 ...
    ]= extract_kinmodel_parameters(ropod_kinmodel_param_vec);

Fxi = (tl/rW1_1+tr/rW1_2);
Fyi = (tr/rW1_2-tl/rW1_1)*(d_w/(2*s_w));
theta = atan2(Fyi,Fxi);

Fsize = abs(Fyi);
if Fsize> Fthr
   sc = (1+(kmax-1)*abs( sin(theta)) );
else
    sc = 1;
end

avg_t = (tr+tl)/2;
diff_t = (tr-tl)/2;
tl_out = avg_t-sc*diff_t;
tr_out = avg_t+sc*diff_t;

if(abs(tl_out)>tau_max && abs(tl_out)>abs(tr_out))
    sc = tau_max/abs(tl_out);
    tl_out = sc*tl_out;
    tr_out = sc*tr_out;
end

if(abs(tr_out)>tau_max && abs(tr_out)>abs(tl_out))
    sc = tau_max/abs(tr_out);
    tl_out = sc*tl_out;
    tr_out = sc*tr_out;
end

== matlab function ROPOD_Control_WheelsRL_Code_GEN/RopodTorqueDistribution_/Own Constrainst Calculator ==
  data: enable_local_robot output; ropod_kinmodel_param_vec input; tau_max input; constraints_local_robot output; ena_sw input
function [enable_local_robot, constraints_local_robot ] = calculateConstraints(ropod_kinmodel_param_vec, tau_max, ena_sw)
persistent ena_sw_prev;
persistent tau_max_prev;
persistent constraints_local_robot_internal;
persistent enable_local_robot_internal;

if isempty(ena_sw_prev)
    ena_sw_prev = zeros(size(ena_sw));
    tau_max_prev = 0;
    constraints_local_robot_internal = zeros(8,1);
    enable_local_robot_internal = 0;
end

Nwheels = length(ena_sw);

ena_sw_new = 0;
for i_ena = 1: Nwheels
    if(ena_sw_prev(i_ena)~=ena_sw(i_ena))
        ena_sw_new = 1;
        break;
    end
end

if(   ena_sw_new~=0 ...
   || tau_max_prev ~= tau_max)
    
    [  rW1_1,rW1_2,rW1_3,rW1_4,rW2_1,rW2_2,rW2_3,rW2_4,...
        s_w,...
        d_w, ...
        CW1_1,CW1_2,CW1_3,CW1_4,CW2_1,CW2_2,CW2_3,CW2_4 ...
        ]= extract_kinmodel_parameters(ropod_kinmodel_param_vec);
    
    rw = rW1_1;
    % Conservtaive approach use only forward force of smartwheel, which is
    % the smallest of all directions. In any case forces in other directions
    % last little since the wheels will align in the direction of movement.
    
    Fsw_max = 2*tau_max/rw;
    
    
    CW = [[CW1_1 ; CW2_1], [CW1_2 ; CW2_2], [CW1_3 ; CW2_3], [CW1_4 ; CW2_4]];
    
    
    %% First compute the matrix from v to W_wh
    
    % Gi = zeros([2 3]);
    G = zeros(2*Nwheels,3);
    M = zeros(2*Nwheels,2*Nwheels);
    
    for i=1:Nwheels
        % To obtain pivot velocities in Robot coordinates, add vectors of
        % translations and movement due to angular velocity.
        Gi = [1 0 -CW(2,i);
            0 1  CW(1,i)];
        
        G(2*i-1:2*i,:) = Gi;
        M(2*i-1:2*i,2*i-1:2*i)=diag([ena_sw(i) ena_sw(i)]);
    end
    
    GtS = (M*G)'*eye(8);
    
    if(sum(ena_sw)<2)
        enable_local_robot_internal = 0;
        Fx_max_ropod = 0;
        Fy_max_ropod = 0;
    else
        enable_local_robot_internal = 1;
        % Compute Force at pivots to actuate 1N in x at the ropod. Then scale up.
        Fpiv1Nx = pinv(GtS)*[1 0 0]';
        Fx_max_ropod = Fsw_max/max(abs(Fpiv1Nx));
        Fpiv1Ny = pinv(GtS)*[0 1 0]';
        Fy_max_ropod = Fsw_max/max(abs(Fpiv1Ny));
    end
    
    
    % Eight elements with x,y position of constraint
    constraints_local_robot_internal = ...
        [
        Fx_max_ropod,   0, ...
        0,              Fy_max_ropod , ...
        -Fx_max_ropod,  0, ...
        0,             -Fy_max_ropod  ...
        ]';
    
end

ena_sw_prev = ena_sw;
tau_max_prev = tau_max;

constraints_local_robot = constraints_local_robot_internal;
enable_local_robot = enable_local_robot_internal;



end

== matlab function ROPOD_Control_WheelsRL_Code_GEN/RopodTorqueDistribution_/ROPOD 4SW/ROPOD_4Wheel_sens_own_vel_filter/Glitch removal + LP filter/Remove_glitches1 ==
  data: vel input; Ts input; encoder input; encoder_out output
function encoder_out  = remove_glitches(vel, Ts, encoder)

persistent last_valid_encoder;
persistent invalid_cnt;

if(isempty(last_valid_encoder))
    last_valid_encoder = encoder;
    invalid_cnt = 0;
end

if abs( (last_valid_encoder-encoder)/Ts ) > 50 % maximum expected velocity rad/sec (2.5 m/s)
    encoder_out = last_valid_encoder + vel*Ts;    
    invalid_cnt = invalid_cnt +1;
else
    encoder_out = encoder;
end

if invalid_cnt>1 
    invalid_cnt = 0;
    encoder_out = encoder;
end

last_valid_encoder = encoder_out;

== matlab function ROPOD_Control_WheelsRL_Code_GEN/RopodTorqueDistribution_/ROPOD 4SW/ROPOD_4Wheel_sens_own_vel_filter/Glitch removal + LP filter1/Remove_glitches1 ==
  data: vel input; Ts input; encoder input; encoder_out output
function encoder_out  = remove_glitches(vel, Ts, encoder)

persistent last_valid_encoder;
persistent invalid_cnt;

if(isempty(last_valid_encoder))
    last_valid_encoder = encoder;
    invalid_cnt = 0;
end

if abs( (last_valid_encoder-encoder)/Ts ) > 50 % maximum expected velocity rad/sec (2.5 m/s)
    encoder_out = last_valid_encoder + vel*Ts;    
    invalid_cnt = invalid_cnt +1;
else
    encoder_out = encoder;
end

if invalid_cnt>1 
    invalid_cnt = 0;
    encoder_out = encoder;
end

last_valid_encoder = encoder_out;

== matlab function ROPOD_Control_WheelsRL_Code_GEN/RopodTorqueDistribution_/ROPOD 4SW/ROPOD_4Wheel_sens_own_vel_filter/Glitch removal + LP filter10/Remove_glitches1 ==
  data: vel input; Ts input; encoder input; encoder_out output
function encoder_out  = remove_glitches(vel, Ts, encoder)

persistent last_valid_encoder;
persistent invalid_cnt;

if(isempty(last_valid_encoder))
    last_valid_encoder = encoder;
    invalid_cnt = 0;
end

if abs( (last_valid_encoder-encoder)/Ts ) > 50 % maximum expected velocity rad/sec (2.5 m/s)
    encoder_out = last_valid_encoder + vel*Ts;    
    invalid_cnt = invalid_cnt +1;
else
    encoder_out = encoder;
end

if invalid_cnt>1 
    invalid_cnt = 0;
    encoder_out = encoder;
end

last_valid_encoder = encoder_out;

== matlab function ROPOD_Control_WheelsRL_Code_GEN/RopodTorqueDistribution_/ROPOD 4SW/ROPOD_4Wheel_sens_own_vel_filter/Glitch removal + LP filter11/Remove_glitches1 ==
  data: vel input; Ts input; encoder input; encoder_out output
function encoder_out  = remove_glitches(vel, Ts, encoder)

persistent last_valid_encoder;
persistent invalid_cnt;

if(isempty(last_valid_encoder))
    last_valid_encoder = encoder;
    invalid_cnt = 0;
end

if abs( (last_valid_encoder-encoder)/Ts ) > 50 % maximum expected velocity rad/sec (2.5 m/s)
    encoder_out = last_valid_encoder + vel*Ts;    
    invalid_cnt = invalid_cnt +1;
else
    encoder_out = encoder;
end

if invalid_cnt>1 
    invalid_cnt = 0;
    encoder_out = encoder;
end

last_valid_encoder = encoder_out;

== matlab function ROPOD_Control_WheelsRL_Code_GEN/RopodTorqueDistribution_/ROPOD 4SW/ROPOD_4Wheel_sens_own_vel_filter/Glitch removal + LP filter2/Remove_glitches1 ==
  data: vel input; Ts input; encoder input; encoder_out output
function encoder_out  = remove_glitches(vel, Ts, encoder)

persistent last_valid_encoder;
persistent invalid_cnt;

if(isempty(last_valid_encoder))
    last_valid_encoder = encoder;
    invalid_cnt = 0;
end

if abs( (last_valid_encoder-encoder)/Ts ) > 50 % maximum expected velocity rad/sec (2.5 m/s)
    encoder_out = last_valid_encoder + vel*Ts;    
    invalid_cnt = invalid_cnt +1;
else
    encoder_out = encoder;
end

if invalid_cnt>1 
    invalid_cnt = 0;
    encoder_out = encoder;
end

last_valid_encoder = encoder_out;
